simulink model "model"  (R2024a)
settings: Solver=FixedStepAuto  StartTime=0.0  StopTime=6  FixedStep=0.001  RelTol=1e-3
undefined symbols (not defined in the file): K, T1, T2
settings Model: Creator=Professional  LastModifiedBy=Professional

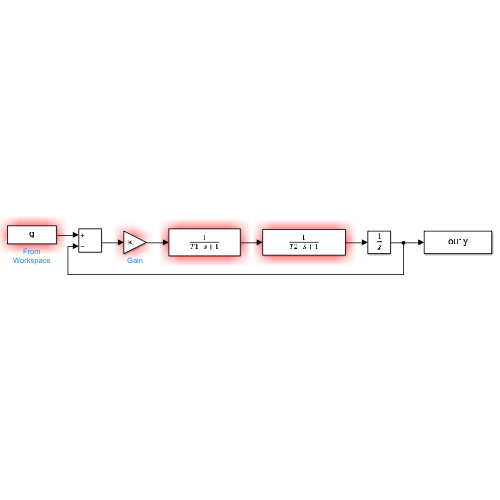
[thumbnail: Simulink's stored preview of the top-level diagram]
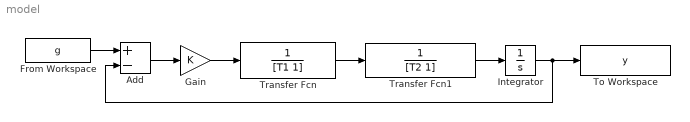
== system model ==
  Add : Sum  Inputs=+-
  From Workspace : FromWorkspace  VariableName=g
  Gain : Gain  Gain=K
  Integrator : Integrator
  To Workspace : ToWorkspace  VariableName=y  SaveFormat=Timeseries  SampleTime=-1
  Transfer Fcn : TransferFcn  Denominator=[T1 1]
  Transfer Fcn1 : TransferFcn  Denominator=[T2 1]
  wires:
  From Workspace/1 -> Add/1
  Add/1 -> Gain/1
  Gain/1 -> Transfer Fcn/1
  Transfer Fcn/1 -> Transfer Fcn1/1
  Transfer Fcn1/1 -> Integrator/1
  Integrator/1 -> Add/2, To Workspace/1
